simulink model "pattern3x3_testing_2023v1"  (R2023a)
settings: Solver=FixedStepAuto  StartTime=0.0  StopTime=2  FixedStep=0.000005  RelTol=1e-3
values from neighbouring files (symbols this model uses):
  test_pattern = load('Pattern4_test.CSV')    [model_setup_test.m]
  Th_control_time2 = 0.02    [model_setup4.m]    (also in model_setup_test.m = 2)
  Th_minus_count2 = 10    [model_setup4.m]    (also in model_setup_test.m = 5)
  Th_plus_count2 = 20    [model_setup4.m]    (also in model_setup_test.m)
libraries: simulink x1
(part 4 of 4)

== system pattern3x3_testing_2023v1/Synapse30/Spike_gererator ==
  "Spike " : Inport
  AND : Logic  IconShape=distinctive  AllPortsSameDT=off  OutDataTypeStr=boolean
  Delay : Delay  DelayLength=1  SampleTime=0.00001
  NOT : Logic  Operator=NOT  IconShape=distinctive  AllPortsSameDT=off  OutDataTypeStr=boolean
  Spike_out : Outport  VectorParamsAs1DForOutWhenUnconnected=off
  wires:
  "Spike "/1 -> NOT/1, AND/1
  AND/1 -> Spike_out/1
  Delay/1 -> AND/2
  NOT/1 -> Delay/1

== system pattern3x3_testing_2023v1/Synapse31/Spike_gererator ==
  "Spike " : Inport
  AND : Logic  IconShape=distinctive  AllPortsSameDT=off  OutDataTypeStr=boolean
  Delay : Delay  DelayLength=1  SampleTime=0.00001
  NOT : Logic  Operator=NOT  IconShape=distinctive  AllPortsSameDT=off  OutDataTypeStr=boolean
  Spike_out : Outport  VectorParamsAs1DForOutWhenUnconnected=off
  wires:
  "Spike "/1 -> NOT/1, AND/1
  AND/1 -> Spike_out/1
  Delay/1 -> AND/2
  NOT/1 -> Delay/1

== system pattern3x3_testing_2023v1/Synapse32/Spike_gererator ==
  "Spike " : Inport
  AND : Logic  IconShape=distinctive  AllPortsSameDT=off  OutDataTypeStr=boolean
  Delay : Delay  DelayLength=1  SampleTime=0.00001
  NOT : Logic  Operator=NOT  IconShape=distinctive  AllPortsSameDT=off  OutDataTypeStr=boolean
  Spike_out : Outport  VectorParamsAs1DForOutWhenUnconnected=off
  wires:
  "Spike "/1 -> NOT/1, AND/1
  AND/1 -> Spike_out/1
  Delay/1 -> AND/2
  NOT/1 -> Delay/1

== system pattern3x3_testing_2023v1/Synapse33/Spike_gererator ==
  "Spike " : Inport
  AND : Logic  IconShape=distinctive  AllPortsSameDT=off  OutDataTypeStr=boolean
  Delay : Delay  DelayLength=1  SampleTime=0.00001
  NOT : Logic  Operator=NOT  IconShape=distinctive  AllPortsSameDT=off  OutDataTypeStr=boolean
  Spike_out : Outport  VectorParamsAs1DForOutWhenUnconnected=off
  wires:
  "Spike "/1 -> NOT/1, AND/1
  AND/1 -> Spike_out/1
  Delay/1 -> AND/2
  NOT/1 -> Delay/1

== system pattern3x3_testing_2023v1/Synapse34/Spike_gererator ==
  "Spike " : Inport
  AND : Logic  IconShape=distinctive  AllPortsSameDT=off  OutDataTypeStr=boolean
  Delay : Delay  DelayLength=1  SampleTime=0.00001
  NOT : Logic  Operator=NOT  IconShape=distinctive  AllPortsSameDT=off  OutDataTypeStr=boolean
  Spike_out : Outport  VectorParamsAs1DForOutWhenUnconnected=off
  wires:
  "Spike "/1 -> NOT/1, AND/1
  AND/1 -> Spike_out/1
  Delay/1 -> AND/2
  NOT/1 -> Delay/1

== system pattern3x3_testing_2023v1/Synapse35/Spike_gererator ==
  "Spike " : Inport
  AND : Logic  IconShape=distinctive  AllPortsSameDT=off  OutDataTypeStr=boolean
  Delay : Delay  DelayLength=1  SampleTime=0.00001
  NOT : Logic  Operator=NOT  IconShape=distinctive  AllPortsSameDT=off  OutDataTypeStr=boolean
  Spike_out : Outport  VectorParamsAs1DForOutWhenUnconnected=off
  wires:
  "Spike "/1 -> NOT/1, AND/1
  AND/1 -> Spike_out/1
  Delay/1 -> AND/2
  NOT/1 -> Delay/1

== system pattern3x3_testing_2023v1/Synapse36/Spike_gererator ==
  "Spike " : Inport
  AND : Logic  IconShape=distinctive  AllPortsSameDT=off  OutDataTypeStr=boolean
  Delay : Delay  DelayLength=1  SampleTime=0.00001
  NOT : Logic  Operator=NOT  IconShape=distinctive  AllPortsSameDT=off  OutDataTypeStr=boolean
  Spike_out : Outport  VectorParamsAs1DForOutWhenUnconnected=off
  wires:
  "Spike "/1 -> NOT/1, AND/1
  AND/1 -> Spike_out/1
  Delay/1 -> AND/2
  NOT/1 -> Delay/1

== system pattern3x3_testing_2023v1/Synapse4/Spike_gererator ==
  "Spike " : Inport
  AND : Logic  IconShape=distinctive  AllPortsSameDT=off  OutDataTypeStr=boolean
  Delay : Delay  DelayLength=1  SampleTime=0.00001
  NOT : Logic  Operator=NOT  IconShape=distinctive  AllPortsSameDT=off  OutDataTypeStr=boolean
  Spike_out : Outport  VectorParamsAs1DForOutWhenUnconnected=off
  wires:
  "Spike "/1 -> NOT/1, AND/1
  AND/1 -> Spike_out/1
  Delay/1 -> AND/2
  NOT/1 -> Delay/1

== system pattern3x3_testing_2023v1/Synapse5/Spike_gererator ==
  "Spike " : Inport
  AND : Logic  IconShape=distinctive  AllPortsSameDT=off  OutDataTypeStr=boolean
  Delay : Delay  DelayLength=1  SampleTime=0.00001
  NOT : Logic  Operator=NOT  IconShape=distinctive  AllPortsSameDT=off  OutDataTypeStr=boolean
  Spike_out : Outport  VectorParamsAs1DForOutWhenUnconnected=off
  wires:
  "Spike "/1 -> NOT/1, AND/1
  AND/1 -> Spike_out/1
  Delay/1 -> AND/2
  NOT/1 -> Delay/1

== system pattern3x3_testing_2023v1/Synapse6/Spike_gererator ==
  "Spike " : Inport
  AND : Logic  IconShape=distinctive  AllPortsSameDT=off  OutDataTypeStr=boolean
  Delay : Delay  DelayLength=1  SampleTime=0.00001
  NOT : Logic  Operator=NOT  IconShape=distinctive  AllPortsSameDT=off  OutDataTypeStr=boolean
  Spike_out : Outport  VectorParamsAs1DForOutWhenUnconnected=off
  wires:
  "Spike "/1 -> NOT/1, AND/1
  AND/1 -> Spike_out/1
  Delay/1 -> AND/2
  NOT/1 -> Delay/1

== system pattern3x3_testing_2023v1/Synapse7/Spike_gererator ==
  "Spike " : Inport
  AND : Logic  IconShape=distinctive  AllPortsSameDT=off  OutDataTypeStr=boolean
  Delay : Delay  DelayLength=1  SampleTime=0.00001
  NOT : Logic  Operator=NOT  IconShape=distinctive  AllPortsSameDT=off  OutDataTypeStr=boolean
  Spike_out : Outport  VectorParamsAs1DForOutWhenUnconnected=off
  wires:
  "Spike "/1 -> NOT/1, AND/1
  AND/1 -> Spike_out/1
  Delay/1 -> AND/2
  NOT/1 -> Delay/1

== system pattern3x3_testing_2023v1/Synapse8/Spike_gererator ==
  "Spike " : Inport
  AND : Logic  IconShape=distinctive  AllPortsSameDT=off  OutDataTypeStr=boolean
  Delay : Delay  DelayLength=1  SampleTime=0.00001
  NOT : Logic  Operator=NOT  IconShape=distinctive  AllPortsSameDT=off  OutDataTypeStr=boolean
  Spike_out : Outport  VectorParamsAs1DForOutWhenUnconnected=off
  wires:
  "Spike "/1 -> NOT/1, AND/1
  AND/1 -> Spike_out/1
  Delay/1 -> AND/2
  NOT/1 -> Delay/1

== system pattern3x3_testing_2023v1/Synapse9/Spike_gererator ==
  "Spike " : Inport
  AND : Logic  IconShape=distinctive  AllPortsSameDT=off  OutDataTypeStr=boolean
  Delay : Delay  DelayLength=1  SampleTime=0.00001
  NOT : Logic  Operator=NOT  IconShape=distinctive  AllPortsSameDT=off  OutDataTypeStr=boolean
  Spike_out : Outport  VectorParamsAs1DForOutWhenUnconnected=off
  wires:
  "Spike "/1 -> NOT/1, AND/1
  AND/1 -> Spike_out/1
  Delay/1 -> AND/2
  NOT/1 -> Delay/1

== system pattern3x3_testing_2023v1/Neuron1/Clock4/Triggered Subsystem1 ==
  In1 : Inport
  Trigger : TriggerPort  VariantControl=Variant
  Constant : Constant
  Sum : Sum  Inputs=|++
  Out1 : Outport  VectorParamsAs1DForOutWhenUnconnected=off
  wires:
  Constant/1 -> Sum/2
  In1/1 -> Sum/1
  Sum/1 -> Out1/1

== system pattern3x3_testing_2023v1/Neuron1/Clock5/Triggered Subsystem1 ==
  In1 : Inport
  Trigger : TriggerPort  VariantControl=Variant
  Constant : Constant
  Sum : Sum  Inputs=|++
  Out1 : Outport  VectorParamsAs1DForOutWhenUnconnected=off
  wires:
  Constant/1 -> Sum/2
  In1/1 -> Sum/1
  Sum/1 -> Out1/1

== system pattern3x3_testing_2023v1/Neuron1/Subsystem3/spike_generator2 ==
  del_th : Inport
  AND : Logic  IconShape=distinctive  AllPortsSameDT=off  OutDataTypeStr=boolean
  Delay1 : Delay  DelayLength=1  SampleTime=0.00001
  NOT : Logic  Operator=NOT  IconShape=distinctive  AllPortsSameDT=off  OutDataTypeStr=boolean
  Product : Product
  del_th_spike : Outport
  wires:
  NOT/1 -> Delay1/1
  AND/1 -> Product/1
  Delay1/1 -> AND/2
  Product/1 -> del_th_spike/1
  del_th/1 -> AND/1, Product/2, NOT/1

== system pattern3x3_testing_2023v1/Neuron2/Clock4/Triggered Subsystem1 ==
  In1 : Inport
  Trigger : TriggerPort  VariantControl=Variant
  Constant : Constant
  Sum : Sum  Inputs=|++
  Out1 : Outport  VectorParamsAs1DForOutWhenUnconnected=off
  wires:
  Constant/1 -> Sum/2
  In1/1 -> Sum/1
  Sum/1 -> Out1/1

== system pattern3x3_testing_2023v1/Neuron2/Clock5/Triggered Subsystem1 ==
  In1 : Inport
  Trigger : TriggerPort  VariantControl=Variant
  Constant : Constant
  Sum : Sum  Inputs=|++
  Out1 : Outport  VectorParamsAs1DForOutWhenUnconnected=off
  wires:
  Constant/1 -> Sum/2
  In1/1 -> Sum/1
  Sum/1 -> Out1/1

== system pattern3x3_testing_2023v1/Neuron2/Subsystem3/spike_generator2 ==
  del_th : Inport
  AND : Logic  IconShape=distinctive  AllPortsSameDT=off  OutDataTypeStr=boolean
  Delay1 : Delay  DelayLength=1  SampleTime=0.00001
  NOT : Logic  Operator=NOT  IconShape=distinctive  AllPortsSameDT=off  OutDataTypeStr=boolean
  Product : Product
  del_th_spike : Outport
  wires:
  NOT/1 -> Delay1/1
  AND/1 -> Product/1
  Delay1/1 -> AND/2
  Product/1 -> del_th_spike/1
  del_th/1 -> AND/1, Product/2, NOT/1

== system pattern3x3_testing_2023v1/Neuron3/Clock4/Triggered Subsystem1 ==
  In1 : Inport
  Trigger : TriggerPort  VariantControl=Variant
  Constant : Constant
  Sum : Sum  Inputs=|++
  Out1 : Outport  VectorParamsAs1DForOutWhenUnconnected=off
  wires:
  Constant/1 -> Sum/2
  In1/1 -> Sum/1
  Sum/1 -> Out1/1

== system pattern3x3_testing_2023v1/Neuron3/Clock5/Triggered Subsystem1 ==
  In1 : Inport
  Trigger : TriggerPort  VariantControl=Variant
  Constant : Constant
  Sum : Sum  Inputs=|++
  Out1 : Outport  VectorParamsAs1DForOutWhenUnconnected=off
  wires:
  Constant/1 -> Sum/2
  In1/1 -> Sum/1
  Sum/1 -> Out1/1

== system pattern3x3_testing_2023v1/Neuron3/Subsystem3/spike_generator2 ==
  del_th : Inport
  AND : Logic  IconShape=distinctive  AllPortsSameDT=off  OutDataTypeStr=boolean
  Delay1 : Delay  DelayLength=1  SampleTime=0.00001
  NOT : Logic  Operator=NOT  IconShape=distinctive  AllPortsSameDT=off  OutDataTypeStr=boolean
  Product : Product
  del_th_spike : Outport
  wires:
  NOT/1 -> Delay1/1
  AND/1 -> Product/1
  Delay1/1 -> AND/2
  Product/1 -> del_th_spike/1
  del_th/1 -> AND/1, Product/2, NOT/1

== system pattern3x3_testing_2023v1/Neuron4/Clock4/Triggered Subsystem1 ==
  In1 : Inport
  Trigger : TriggerPort  VariantControl=Variant
  Constant : Constant
  Sum : Sum  Inputs=|++
  Out1 : Outport  VectorParamsAs1DForOutWhenUnconnected=off
  wires:
  Constant/1 -> Sum/2
  In1/1 -> Sum/1
  Sum/1 -> Out1/1

== system pattern3x3_testing_2023v1/Neuron4/Clock5/Triggered Subsystem1 ==
  In1 : Inport
  Trigger : TriggerPort  VariantControl=Variant
  Constant : Constant
  Sum : Sum  Inputs=|++
  Out1 : Outport  VectorParamsAs1DForOutWhenUnconnected=off
  wires:
  Constant/1 -> Sum/2
  In1/1 -> Sum/1
  Sum/1 -> Out1/1

== system pattern3x3_testing_2023v1/Neuron4/Subsystem3/spike_generator2 ==
  del_th : Inport
  AND : Logic  IconShape=distinctive  AllPortsSameDT=off  OutDataTypeStr=boolean
  Delay1 : Delay  DelayLength=1  SampleTime=0.00001
  NOT : Logic  Operator=NOT  IconShape=distinctive  AllPortsSameDT=off  OutDataTypeStr=boolean
  Product : Product
  del_th_spike : Outport
  wires:
  NOT/1 -> Delay1/1
  AND/1 -> Product/1
  Delay1/1 -> AND/2
  Product/1 -> del_th_spike/1
  del_th/1 -> AND/1, Product/2, NOT/1

== system pattern3x3_testing_2023v1/Neuron5/Clock4/Triggered Subsystem1 ==
  In1 : Inport
  Trigger : TriggerPort  VariantControl=Variant
  Constant : Constant
  Sum : Sum  Inputs=|++
  Out1 : Outport  VectorParamsAs1DForOutWhenUnconnected=off
  wires:
  Constant/1 -> Sum/2
  In1/1 -> Sum/1
  Sum/1 -> Out1/1

== system pattern3x3_testing_2023v1/Neuron5/Clock5/Triggered Subsystem1 ==
  In1 : Inport
  Trigger : TriggerPort  VariantControl=Variant
  Constant : Constant
  Sum : Sum  Inputs=|++
  Out1 : Outport  VectorParamsAs1DForOutWhenUnconnected=off
  wires:
  Constant/1 -> Sum/2
  In1/1 -> Sum/1
  Sum/1 -> Out1/1

== system pattern3x3_testing_2023v1/Neuron5/Subsystem3/spike_generator2 ==
  del_th : Inport
  AND : Logic  IconShape=distinctive  AllPortsSameDT=off  OutDataTypeStr=boolean
  Delay1 : Delay  DelayLength=1  SampleTime=0.00001
  NOT : Logic  Operator=NOT  IconShape=distinctive  AllPortsSameDT=off  OutDataTypeStr=boolean
  Product : Product
  del_th_spike : Outport
  wires:
  NOT/1 -> Delay1/1
  AND/1 -> Product/1
  Delay1/1 -> AND/2
  Product/1 -> del_th_spike/1
  del_th/1 -> AND/1, Product/2, NOT/1

== system pattern3x3_testing_2023v1/Neuron6/Clock4/Triggered Subsystem1 ==
  In1 : Inport
  Trigger : TriggerPort  VariantControl=Variant
  Constant : Constant
  Sum : Sum  Inputs=|++
  Out1 : Outport  VectorParamsAs1DForOutWhenUnconnected=off
  wires:
  Constant/1 -> Sum/2
  In1/1 -> Sum/1
  Sum/1 -> Out1/1

== system pattern3x3_testing_2023v1/Neuron6/Clock5/Triggered Subsystem1 ==
  In1 : Inport
  Trigger : TriggerPort  VariantControl=Variant
  Constant : Constant
  Sum : Sum  Inputs=|++
  Out1 : Outport  VectorParamsAs1DForOutWhenUnconnected=off
  wires:
  Constant/1 -> Sum/2
  In1/1 -> Sum/1
  Sum/1 -> Out1/1

== system pattern3x3_testing_2023v1/Neuron6/Subsystem3/spike_generator2 ==
  del_th : Inport
  AND : Logic  IconShape=distinctive  AllPortsSameDT=off  OutDataTypeStr=boolean
  Delay1 : Delay  DelayLength=1  SampleTime=0.00001
  NOT : Logic  Operator=NOT  IconShape=distinctive  AllPortsSameDT=off  OutDataTypeStr=boolean
  Product : Product
  del_th_spike : Outport
  wires:
  NOT/1 -> Delay1/1
  AND/1 -> Product/1
  Delay1/1 -> AND/2
  Product/1 -> del_th_spike/1
  del_th/1 -> AND/1, Product/2, NOT/1

== system pattern3x3_testing_2023v1/Neuron7/Clock4/Triggered Subsystem1 ==
  In1 : Inport
  Trigger : TriggerPort  VariantControl=Variant
  Constant : Constant
  Sum : Sum  Inputs=|++
  Out1 : Outport  VectorParamsAs1DForOutWhenUnconnected=off
  wires:
  Constant/1 -> Sum/2
  In1/1 -> Sum/1
  Sum/1 -> Out1/1

== system pattern3x3_testing_2023v1/Neuron7/Clock5/Triggered Subsystem1 ==
  In1 : Inport
  Trigger : TriggerPort  VariantControl=Variant
  Constant : Constant
  Sum : Sum  Inputs=|++
  Out1 : Outport  VectorParamsAs1DForOutWhenUnconnected=off
  wires:
  Constant/1 -> Sum/2
  In1/1 -> Sum/1
  Sum/1 -> Out1/1

== system pattern3x3_testing_2023v1/Neuron7/Subsystem3/spike_generator2 ==
  del_th : Inport
  AND : Logic  IconShape=distinctive  AllPortsSameDT=off  OutDataTypeStr=boolean
  Delay1 : Delay  DelayLength=1  SampleTime=0.00001
  NOT : Logic  Operator=NOT  IconShape=distinctive  AllPortsSameDT=off  OutDataTypeStr=boolean
  Product : Product
  del_th_spike : Outport
  wires:
  NOT/1 -> Delay1/1
  AND/1 -> Product/1
  Delay1/1 -> AND/2
  Product/1 -> del_th_spike/1
  del_th/1 -> AND/1, Product/2, NOT/1

== system pattern3x3_testing_2023v1/Neuron8/Clock4/Triggered Subsystem1 ==
  In1 : Inport
  Trigger : TriggerPort  VariantControl=Variant
  Constant : Constant
  Sum : Sum  Inputs=|++
  Out1 : Outport  VectorParamsAs1DForOutWhenUnconnected=off
  wires:
  Constant/1 -> Sum/2
  In1/1 -> Sum/1
  Sum/1 -> Out1/1

== system pattern3x3_testing_2023v1/Neuron8/Clock5/Triggered Subsystem1 ==
  In1 : Inport
  Trigger : TriggerPort  VariantControl=Variant
  Constant : Constant
  Sum : Sum  Inputs=|++
  Out1 : Outport  VectorParamsAs1DForOutWhenUnconnected=off
  wires:
  Constant/1 -> Sum/2
  In1/1 -> Sum/1
  Sum/1 -> Out1/1

== system pattern3x3_testing_2023v1/Neuron8/Subsystem3/spike_generator2 ==
  del_th : Inport
  AND : Logic  IconShape=distinctive  AllPortsSameDT=off  OutDataTypeStr=boolean
  Delay1 : Delay  DelayLength=1  SampleTime=0.00001
  NOT : Logic  Operator=NOT  IconShape=distinctive  AllPortsSameDT=off  OutDataTypeStr=boolean
  Product : Product
  del_th_spike : Outport
  wires:
  NOT/1 -> Delay1/1
  AND/1 -> Product/1
  Delay1/1 -> AND/2
  Product/1 -> del_th_spike/1
  del_th/1 -> AND/1, Product/2, NOT/1

== system pattern3x3_testing_2023v1/Neuron9/Clock4/Triggered Subsystem1 ==
  In1 : Inport
  Trigger : TriggerPort  VariantControl=Variant
  Constant : Constant
  Sum : Sum  Inputs=|++
  Out1 : Outport  VectorParamsAs1DForOutWhenUnconnected=off
  wires:
  Constant/1 -> Sum/2
  In1/1 -> Sum/1
  Sum/1 -> Out1/1

== system pattern3x3_testing_2023v1/Neuron9/Clock5/Triggered Subsystem1 ==
  In1 : Inport
  Trigger : TriggerPort  VariantControl=Variant
  Constant : Constant
  Sum : Sum  Inputs=|++
  Out1 : Outport  VectorParamsAs1DForOutWhenUnconnected=off
  wires:
  Constant/1 -> Sum/2
  In1/1 -> Sum/1
  Sum/1 -> Out1/1

== system pattern3x3_testing_2023v1/Neuron9/Subsystem3/spike_generator2 ==
  del_th : Inport
  AND : Logic  IconShape=distinctive  AllPortsSameDT=off  OutDataTypeStr=boolean
  Delay1 : Delay  DelayLength=1  SampleTime=0.00001
  NOT : Logic  Operator=NOT  IconShape=distinctive  AllPortsSameDT=off  OutDataTypeStr=boolean
  Product : Product
  del_th_spike : Outport
  wires:
  NOT/1 -> Delay1/1
  AND/1 -> Product/1
  Delay1/1 -> AND/2
  Product/1 -> del_th_spike/1
  del_th/1 -> AND/1, Product/2, NOT/1

== system pattern3x3_testing_2023v1/Post_Neuron1/Clock4/Triggered Subsystem1 ==
  In1 : Inport
  Trigger : TriggerPort  VariantControl=Variant
  Constant : Constant
  Sum : Sum  Inputs=|++
  Out1 : Outport  VectorParamsAs1DForOutWhenUnconnected=off
  wires:
  Constant/1 -> Sum/2
  In1/1 -> Sum/1
  Sum/1 -> Out1/1

== system pattern3x3_testing_2023v1/Post_Neuron1/Clock6/Triggered Subsystem1 ==
  In1 : Inport
  Trigger : TriggerPort  VariantControl=Variant
  Constant : Constant
  Sum : Sum  Inputs=|++
  Out1 : Outport  VectorParamsAs1DForOutWhenUnconnected=off
  wires:
  Constant/1 -> Sum/2
  In1/1 -> Sum/1
  Sum/1 -> Out1/1

== system pattern3x3_testing_2023v1/Post_Neuron1/Subsystem3/spike_generator2 ==
  del_th : Inport
  AND : Logic  IconShape=distinctive  AllPortsSameDT=off  OutDataTypeStr=boolean
  Delay1 : Delay  DelayLength=1  SampleTime=0.00001
  NOT : Logic  Operator=NOT  IconShape=distinctive  AllPortsSameDT=off  OutDataTypeStr=boolean
  Product : Product
  del_th_spike : Outport
  wires:
  NOT/1 -> Delay1/1
  AND/1 -> Product/1
  Delay1/1 -> AND/2
  Product/1 -> del_th_spike/1
  del_th/1 -> AND/1, Product/2, NOT/1

== system pattern3x3_testing_2023v1/Post_Neuron2/Clock4/Triggered Subsystem1 ==
  In1 : Inport
  Trigger : TriggerPort  VariantControl=Variant
  Constant : Constant
  Sum : Sum  Inputs=|++
  Out1 : Outport  VectorParamsAs1DForOutWhenUnconnected=off
  wires:
  Constant/1 -> Sum/2
  In1/1 -> Sum/1
  Sum/1 -> Out1/1

== system pattern3x3_testing_2023v1/Post_Neuron2/Clock6/Triggered Subsystem1 ==
  In1 : Inport
  Trigger : TriggerPort  VariantControl=Variant
  Constant : Constant
  Sum : Sum  Inputs=|++
  Out1 : Outport  VectorParamsAs1DForOutWhenUnconnected=off
  wires:
  Constant/1 -> Sum/2
  In1/1 -> Sum/1
  Sum/1 -> Out1/1

== system pattern3x3_testing_2023v1/Post_Neuron2/Subsystem3/spike_generator2 ==
  del_th : Inport
  AND : Logic  IconShape=distinctive  AllPortsSameDT=off  OutDataTypeStr=boolean
  Delay1 : Delay  DelayLength=1  SampleTime=0.00001
  NOT : Logic  Operator=NOT  IconShape=distinctive  AllPortsSameDT=off  OutDataTypeStr=boolean
  Product : Product
  del_th_spike : Outport
  wires:
  NOT/1 -> Delay1/1
  AND/1 -> Product/1
  Delay1/1 -> AND/2
  Product/1 -> del_th_spike/1
  del_th/1 -> AND/1, Product/2, NOT/1

== system pattern3x3_testing_2023v1/Post_Neuron3/Clock4/Triggered Subsystem1 ==
  In1 : Inport
  Trigger : TriggerPort  VariantControl=Variant
  Constant : Constant
  Sum : Sum  Inputs=|++
  Out1 : Outport  VectorParamsAs1DForOutWhenUnconnected=off
  wires:
  Constant/1 -> Sum/2
  In1/1 -> Sum/1
  Sum/1 -> Out1/1

== system pattern3x3_testing_2023v1/Post_Neuron3/Clock6/Triggered Subsystem1 ==
  In1 : Inport
  Trigger : TriggerPort  VariantControl=Variant
  Constant : Constant
  Sum : Sum  Inputs=|++
  Out1 : Outport  VectorParamsAs1DForOutWhenUnconnected=off
  wires:
  Constant/1 -> Sum/2
  In1/1 -> Sum/1
  Sum/1 -> Out1/1

== system pattern3x3_testing_2023v1/Post_Neuron3/Subsystem3/spike_generator2 ==
  del_th : Inport
  AND : Logic  IconShape=distinctive  AllPortsSameDT=off  OutDataTypeStr=boolean
  Delay1 : Delay  DelayLength=1  SampleTime=0.00001
  NOT : Logic  Operator=NOT  IconShape=distinctive  AllPortsSameDT=off  OutDataTypeStr=boolean
  Product : Product
  del_th_spike : Outport
  wires:
  NOT/1 -> Delay1/1
  AND/1 -> Product/1
  Delay1/1 -> AND/2
  Product/1 -> del_th_spike/1
  del_th/1 -> AND/1, Product/2, NOT/1

== system pattern3x3_testing_2023v1/Post_Neuron4/Clock4/Triggered Subsystem1 ==
  In1 : Inport
  Trigger : TriggerPort  VariantControl=Variant
  Constant : Constant
  Sum : Sum  Inputs=|++
  Out1 : Outport  VectorParamsAs1DForOutWhenUnconnected=off
  wires:
  Constant/1 -> Sum/2
  In1/1 -> Sum/1
  Sum/1 -> Out1/1

== system pattern3x3_testing_2023v1/Post_Neuron4/Clock6/Triggered Subsystem1 ==
  In1 : Inport
  Trigger : TriggerPort  VariantControl=Variant
  Constant : Constant
  Sum : Sum  Inputs=|++
  Out1 : Outport  VectorParamsAs1DForOutWhenUnconnected=off
  wires:
  Constant/1 -> Sum/2
  In1/1 -> Sum/1
  Sum/1 -> Out1/1

== system pattern3x3_testing_2023v1/Post_Neuron4/Subsystem3/spike_generator2 ==
  del_th : Inport
  AND : Logic  IconShape=distinctive  AllPortsSameDT=off  OutDataTypeStr=boolean
  Delay1 : Delay  DelayLength=1  SampleTime=0.00001
  NOT : Logic  Operator=NOT  IconShape=distinctive  AllPortsSameDT=off  OutDataTypeStr=boolean
  Product : Product
  del_th_spike : Outport
  wires:
  NOT/1 -> Delay1/1
  AND/1 -> Product/1
  Delay1/1 -> AND/2
  Product/1 -> del_th_spike/1
  del_th/1 -> AND/1, Product/2, NOT/1

== matlab function pattern3x3_testing_2023v1/Neuron4/MATLAB Function3 ==
  data: u input; y output
function y = fcn(u)

if u>=0
    y=1;
else
    y=0;
end

== matlab function pattern3x3_testing_2023v1/Neuron4/MATLAB Function4 ==
  data: membrane_state input; t input; membrane_potential output
function membrane_potential = fcn(membrane_state, t)

membrane_potential = (membrane_state) * (exp(-(t)*0.015));

== matlab function pattern3x3_testing_2023v1/Neuron2/MATLAB Function3 ==
  data: u input; y output
function y = fcn(u)

if u>=0
    y=1;
else
    y=0;
end

== matlab function pattern3x3_testing_2023v1/Neuron4/MATLAB Function5 ==
  data: t input; membrane_state input; membrane_potential output
function membrane_potential = fcn(t, membrane_state)

membrane_potential = (membrane_state) * 2.361128*(exp(-(t)*0.09)-0.6*exp(-(t+1)*0.04)) ;

== matlab function pattern3x3_testing_2023v1/Neuron4/Subsystem3/MATLAB Function ==
  data: u input; y output; min input; max input
function y = fcn(u, min, max)

if u<=min
    y=min;
elseif u>=max
    y=max;
else
    y=u;
end

== matlab function pattern3x3_testing_2023v1/Neuron4/Subsystem3/MATLAB Function2 ==
  data: init_th input; y output; neuron_num input; before_threshold input
function y = fcn(init_th, neuron_num, before_threshold)

persistent n;

if isempty(n)
    n=init_th(neuron_num);
else
    n=before_threshold;
end

y=n;

== matlab function pattern3x3_testing_2023v1/Neuron5/MATLAB Function3 ==
  data: u input; y output
function y = fcn(u)

if u>=0
    y=1;
else
    y=0;
end

== matlab function pattern3x3_testing_2023v1/Neuron5/MATLAB Function4 ==
  data: membrane_state input; t input; membrane_potential output
function membrane_potential = fcn(membrane_state, t)

membrane_potential = (membrane_state) * (exp(-(t)*0.015));

== matlab function pattern3x3_testing_2023v1/Neuron5/MATLAB Function5 ==
  data: t input; membrane_state input; membrane_potential output
function membrane_potential = fcn(t, membrane_state)

membrane_potential = (membrane_state) * 2.361128*(exp(-(t)*0.09)-0.6*exp(-(t+1)*0.04)) ;

== matlab function pattern3x3_testing_2023v1/Neuron5/Subsystem3/MATLAB Function ==
  data: u input; y output; min input; max input
function y = fcn(u, min, max)

if u<=min
    y=min;
elseif u>=max
    y=max;
else
    y=u;
end

== matlab function pattern3x3_testing_2023v1/Neuron5/Subsystem3/MATLAB Function2 ==
  data: init_th input; y output; neuron_num input; before_threshold input
function y = fcn(init_th, neuron_num, before_threshold)

persistent n;

if isempty(n)
    n=init_th(neuron_num);
else
    n=before_threshold;
end

y=n;

== matlab function pattern3x3_testing_2023v1/Neuron2/MATLAB Function4 ==
  data: membrane_state input; t input; membrane_potential output
function membrane_potential = fcn(membrane_state, t)

membrane_potential = (membrane_state) * (exp(-(t)*0.015));

== matlab function pattern3x3_testing_2023v1/Neuron6/MATLAB Function3 ==
  data: u input; y output
function y = fcn(u)

if u>=0
    y=1;
else
    y=0;
end

== matlab function pattern3x3_testing_2023v1/Neuron6/MATLAB Function4 ==
  data: membrane_state input; t input; membrane_potential output
function membrane_potential = fcn(membrane_state, t)

membrane_potential = (membrane_state) * (exp(-(t)*0.015));

== matlab function pattern3x3_testing_2023v1/Neuron6/MATLAB Function5 ==
  data: t input; membrane_state input; membrane_potential output
function membrane_potential = fcn(t, membrane_state)

membrane_potential = (membrane_state) * 2.361128*(exp(-(t)*0.09)-0.6*exp(-(t+1)*0.04)) ;

== matlab function pattern3x3_testing_2023v1/Post_Neuron2/MATLAB Function3 ==
  data: membrane_state input; t input; membrane_potential output
function membrane_potential = fcn(membrane_state, t)

membrane_potential = (membrane_state) * (exp(-(t)*0.015));

== matlab function pattern3x3_testing_2023v1/Post_Neuron2/MATLAB Function4 ==
  data: t input; membrane_state input; membrane_potential output
function membrane_potential = fcn(t, membrane_state)

membrane_potential = (membrane_state) * 2.361128*(exp(-(t)*0.09)-0.6*exp(-(t+1)*0.04)) ;

== matlab function pattern3x3_testing_2023v1/Post_Neuron2/MATLAB Function7 ==
  data: rc input; lateral_inhibition input; t input; inhibition_potential output
function inhibition_potential = fcn(rc, lateral_inhibition, t)

inhibition_potential = -lateral_inhibition * (exp(-(t)*rc));

== matlab function pattern3x3_testing_2023v1/Post_Neuron2/Subsystem3/MATLAB Function ==
  data: u input; y output; min input; max input
function y = fcn(u, min, max)

if u<=min
    y=min;
elseif u>=max
    y=max;
else
    y=u;
end

== matlab function pattern3x3_testing_2023v1/Post_Neuron2/Subsystem3/MATLAB Function2 ==
  data: init_th input; y output; neuron_num input; before_threshold input
function y = fcn(init_th, neuron_num, before_threshold)

persistent n;

if isempty(n)
    n=init_th(neuron_num);
else
    n=before_threshold;
end

y=n;

== matlab function pattern3x3_testing_2023v1/Post_Neuron3/MATLAB Function1 ==
  data: u input; y output
function y = fcn(u)

if u>=0
    y=1;
else
    y=0;
end

== matlab function pattern3x3_testing_2023v1/Post_Neuron3/MATLAB Function2 ==
  data: u input; y output
function y = fcn(u)
persistent k;
if isempty(k)
    k=0;
elseif u>0
    k=1;
end

y=k;

== matlab function pattern3x3_testing_2023v1/Neuron2/MATLAB Function5 ==
  data: t input; membrane_state input; membrane_potential output
function membrane_potential = fcn(t, membrane_state)

membrane_potential = (membrane_state) * 2.361128*(exp(-(t)*0.09)-0.6*exp(-(t+1)*0.04)) ;

== matlab function pattern3x3_testing_2023v1/Post_Neuron3/MATLAB Function3 ==
  data: membrane_state input; t input; membrane_potential output
function membrane_potential = fcn(membrane_state, t)

membrane_potential = (membrane_state) * (exp(-(t)*0.015));

== matlab function pattern3x3_testing_2023v1/Post_Neuron3/MATLAB Function4 ==
  data: t input; membrane_state input; membrane_potential output
function membrane_potential = fcn(t, membrane_state)

membrane_potential = (membrane_state) * 2.361128*(exp(-(t)*0.09)-0.6*exp(-(t+1)*0.04)) ;

== matlab function pattern3x3_testing_2023v1/Post_Neuron3/MATLAB Function7 ==
  data: rc input; lateral_inhibition input; t input; inhibition_potential output
function inhibition_potential = fcn(rc, lateral_inhibition, t)

inhibition_potential = -lateral_inhibition * (exp(-(t)*rc));

== matlab function pattern3x3_testing_2023v1/Neuron6/Subsystem3/MATLAB Function ==
  data: u input; y output; min input; max input
function y = fcn(u, min, max)

if u<=min
    y=min;
elseif u>=max
    y=max;
else
    y=u;
end

== matlab function pattern3x3_testing_2023v1/Neuron6/Subsystem3/MATLAB Function2 ==
  data: init_th input; y output; neuron_num input; before_threshold input
function y = fcn(init_th, neuron_num, before_threshold)

persistent n;

if isempty(n)
    n=init_th(neuron_num);
else
    n=before_threshold;
end

y=n;

== matlab function pattern3x3_testing_2023v1/Post_Neuron3/Subsystem3/MATLAB Function ==
  data: u input; y output; min input; max input
function y = fcn(u, min, max)

if u<=min
    y=min;
elseif u>=max
    y=max;
else
    y=u;
end

== matlab function pattern3x3_testing_2023v1/Post_Neuron3/Subsystem3/MATLAB Function2 ==
  data: init_th input; y output; neuron_num input; before_threshold input
function y = fcn(init_th, neuron_num, before_threshold)

persistent n;

if isempty(n)
    n=init_th(neuron_num);
else
    n=before_threshold;
end

y=n;

== matlab function pattern3x3_testing_2023v1/Post_Neuron4/MATLAB Function1 ==
  data: u input; y output
function y = fcn(u)

if u>=0
    y=1;
else
    y=0;
end

== matlab function pattern3x3_testing_2023v1/Synapse2/MATLAB Function1 ==
  data: y output; syna_var input; addr input
function y = fcn(syna_var,addr)


   
        y=syna_var(addr);
    

end

== matlab function pattern3x3_testing_2023v1/Synapse3/MATLAB Function1 ==
  data: y output; syna_var input; addr input
function y = fcn(syna_var,addr)


   
        y=syna_var(addr);
    

end

== matlab function pattern3x3_testing_2023v1/Post_Neuron2/MATLAB Function1 ==
  data: u input; y output
function y = fcn(u)

if u>=0
    y=1;
else
    y=0;
end

== matlab function pattern3x3_testing_2023v1/Synapse4/MATLAB Function1 ==
  data: y output; syna_var input; addr input
function y = fcn(syna_var,addr)


   
        y=syna_var(addr);
    

end

== matlab function pattern3x3_testing_2023v1/Synapse5/MATLAB Function1 ==
  data: y output; syna_var input; addr input
function y = fcn(syna_var,addr)


   
        y=syna_var(addr);
    

end

== matlab function pattern3x3_testing_2023v1/Synapse6/MATLAB Function1 ==
  data: y output; syna_var input; addr input
function y = fcn(syna_var,addr)


   
        y=syna_var(addr);
    

end

== matlab function pattern3x3_testing_2023v1/Synapse7/MATLAB Function1 ==
  data: y output; syna_var input; addr input
function y = fcn(syna_var,addr)


   
        y=syna_var(addr);
    

end

== matlab function pattern3x3_testing_2023v1/Synapse8/MATLAB Function1 ==
  data: y output; syna_var input; addr input
function y = fcn(syna_var,addr)


   
        y=syna_var(addr);
    

end

== matlab function pattern3x3_testing_2023v1/Synapse9/MATLAB Function1 ==
  data: y output; syna_var input; addr input
function y = fcn(syna_var,addr)


   
        y=syna_var(addr);
    

end

== matlab function pattern3x3_testing_2023v1/Synapse10/MATLAB Function1 ==
  data: y output; syna_var input; addr input
function y = fcn(syna_var,addr)


   
        y=syna_var(addr);
    

end

== matlab function pattern3x3_testing_2023v1/Synapse11/MATLAB Function1 ==
  data: y output; syna_var input; addr input
function y = fcn(syna_var,addr)


   
        y=syna_var(addr);
    

end

== matlab function pattern3x3_testing_2023v1/Synapse12/MATLAB Function1 ==
  data: y output; syna_var input; addr input
function y = fcn(syna_var,addr)


   
        y=syna_var(addr);
    

end

== matlab function pattern3x3_testing_2023v1/Post_Neuron2/MATLAB Function2 ==
  data: u input; y output
function y = fcn(u)
persistent k;
if isempty(k)
    k=0;
elseif u>0
    k=1;
end

y=k;

== matlab function pattern3x3_testing_2023v1/Synapse13/MATLAB Function1 ==
  data: y output; syna_var input; addr input
function y = fcn(syna_var,addr)


   
        y=syna_var(addr);
    

end

== matlab function pattern3x3_testing_2023v1/Synapse14/MATLAB Function1 ==
  data: y output; syna_var input; addr input
function y = fcn(syna_var,addr)


   
        y=syna_var(addr);
    

end

== matlab function pattern3x3_testing_2023v1/Synapse15/MATLAB Function1 ==
  data: y output; syna_var input; addr input
function y = fcn(syna_var,addr)


   
        y=syna_var(addr);
    

end

== matlab function pattern3x3_testing_2023v1/Synapse16/MATLAB Function1 ==
  data: y output; syna_var input; addr input
function y = fcn(syna_var,addr)


   
        y=syna_var(addr);
    

end

== matlab function pattern3x3_testing_2023v1/Synapse17/MATLAB Function1 ==
  data: y output; syna_var input; addr input
function y = fcn(syna_var,addr)


   
        y=syna_var(addr);
    

end

== matlab function pattern3x3_testing_2023v1/Synapse18/MATLAB Function1 ==
  data: y output; syna_var input; addr input
function y = fcn(syna_var,addr)


   
        y=syna_var(addr);
    

end

== matlab function pattern3x3_testing_2023v1/Synapse19/MATLAB Function1 ==
  data: y output; syna_var input; addr input
function y = fcn(syna_var,addr)


   
        y=syna_var(addr);
    

end

== matlab function pattern3x3_testing_2023v1/Synapse20/MATLAB Function1 ==
  data: y output; syna_var input; addr input
function y = fcn(syna_var,addr)


   
        y=syna_var(addr);
    

end

== matlab function pattern3x3_testing_2023v1/Neuron2/Subsystem3/MATLAB Function ==
  data: u input; y output; min input; max input
function y = fcn(u, min, max)

if u<=min
    y=min;
elseif u>=max
    y=max;
else
    y=u;
end

== matlab function pattern3x3_testing_2023v1/Synapse21/MATLAB Function1 ==
  data: y output; syna_var input; addr input
function y = fcn(syna_var,addr)


   
        y=syna_var(addr);
    

end

== matlab function pattern3x3_testing_2023v1/Synapse22/MATLAB Function1 ==
  data: y output; syna_var input; addr input
function y = fcn(syna_var,addr)


   
        y=syna_var(addr);
    

end

== matlab function pattern3x3_testing_2023v1/Synapse23/MATLAB Function1 ==
  data: y output; syna_var input; addr input
function y = fcn(syna_var,addr)


   
        y=syna_var(addr);
    

end

== matlab function pattern3x3_testing_2023v1/Synapse24/MATLAB Function1 ==
  data: y output; syna_var input; addr input
function y = fcn(syna_var,addr)


   
        y=syna_var(addr);
    

end

== matlab function pattern3x3_testing_2023v1/Synapse25/MATLAB Function1 ==
  data: y output; syna_var input; addr input
function y = fcn(syna_var,addr)


   
        y=syna_var(addr);
    

end

== matlab function pattern3x3_testing_2023v1/Synapse26/MATLAB Function1 ==
  data: y output; syna_var input; addr input
function y = fcn(syna_var,addr)


   
        y=syna_var(addr);
    

end

== matlab function pattern3x3_testing_2023v1/Synapse27/MATLAB Function1 ==
  data: y output; syna_var input; addr input
function y = fcn(syna_var,addr)


   
        y=syna_var(addr);
    

end

== matlab function pattern3x3_testing_2023v1/Synapse28/MATLAB Function1 ==
  data: y output; syna_var input; addr input
function y = fcn(syna_var,addr)


   
        y=syna_var(addr);
    

end

== matlab function pattern3x3_testing_2023v1/Synapse29/MATLAB Function1 ==
  data: y output; syna_var input; addr input
function y = fcn(syna_var,addr)


   
        y=syna_var(addr);
    

end

== matlab function pattern3x3_testing_2023v1/Synapse30/MATLAB Function1 ==
  data: y output; syna_var input; addr input
function y = fcn(syna_var,addr)


   
        y=syna_var(addr);
    

end

== matlab function pattern3x3_testing_2023v1/Synapse31/MATLAB Function1 ==
  data: y output; syna_var input; addr input
function y = fcn(syna_var,addr)


   
        y=syna_var(addr);
    

end

== matlab function pattern3x3_testing_2023v1/Synapse32/MATLAB Function1 ==
  data: y output; syna_var input; addr input
function y = fcn(syna_var,addr)


   
        y=syna_var(addr);
    

end

== matlab function pattern3x3_testing_2023v1/Neuron2/Subsystem3/MATLAB Function2 ==
  data: init_th input; y output; neuron_num input; before_threshold input
function y = fcn(init_th, neuron_num, before_threshold)

persistent n;

if isempty(n)
    n=init_th(neuron_num);
else
    n=before_threshold;
end

y=n;

== matlab function pattern3x3_testing_2023v1/Synapse33/MATLAB Function1 ==
  data: y output; syna_var input; addr input
function y = fcn(syna_var,addr)


   
        y=syna_var(addr);
    

end

== matlab function pattern3x3_testing_2023v1/Synapse34/MATLAB Function1 ==
  data: y output; syna_var input; addr input
function y = fcn(syna_var,addr)


   
        y=syna_var(addr);
    

end

== matlab function pattern3x3_testing_2023v1/Synapse35/MATLAB Function1 ==
  data: y output; syna_var input; addr input
function y = fcn(syna_var,addr)


   
        y=syna_var(addr);
    

end

== matlab function pattern3x3_testing_2023v1/Synapse36/MATLAB Function1 ==
  data: y output; syna_var input; addr input
function y = fcn(syna_var,addr)


   
        y=syna_var(addr);
    

end

== matlab function pattern3x3_testing_2023v1/Post_Neuron4/MATLAB Function2 ==
  data: u input; y output
function y = fcn(u)
persistent k;
if isempty(k)
    k=0;
elseif u>0
    k=1;
end

y=k;

== matlab function pattern3x3_testing_2023v1/Post_Neuron4/MATLAB Function3 ==
  data: membrane_state input; t input; membrane_potential output
function membrane_potential = fcn(membrane_state, t)

membrane_potential = (membrane_state) * (exp(-(t)*0.015));

== matlab function pattern3x3_testing_2023v1/Post_Neuron4/MATLAB Function4 ==
  data: t input; membrane_state input; membrane_potential output
function membrane_potential = fcn(t, membrane_state)

membrane_potential = (membrane_state) * 2.361128*(exp(-(t)*0.09)-0.6*exp(-(t+1)*0.04)) ;

== matlab function pattern3x3_testing_2023v1/Post_Neuron4/MATLAB Function7 ==
  data: rc input; lateral_inhibition input; t input; inhibition_potential output
function inhibition_potential = fcn(rc, lateral_inhibition, t)

inhibition_potential = -lateral_inhibition * (exp(-(t)*rc));

== matlab function pattern3x3_testing_2023v1/Post_Neuron4/Subsystem3/MATLAB Function ==
  data: u input; y output; min input; max input
function y = fcn(u, min, max)

if u<=min
    y=min;
elseif u>=max
    y=max;
else
    y=u;
end

== matlab function pattern3x3_testing_2023v1/Post_Neuron4/Subsystem3/MATLAB Function2 ==
  data: init_th input; y output; neuron_num input; before_threshold input
function y = fcn(init_th, neuron_num, before_threshold)

persistent n;

if isempty(n)
    n=init_th(neuron_num);
else
    n=before_threshold;
end

y=n;

== matlab function pattern3x3_testing_2023v1/Neuron7/MATLAB Function3 ==
  data: u input; y output
function y = fcn(u)

if u>=0
    y=1;
else
    y=0;
end

== matlab function pattern3x3_testing_2023v1/Neuron3/MATLAB Function3 ==
  data: u input; y output
function y = fcn(u)

if u>=0
    y=1;
else
    y=0;
end

== matlab function pattern3x3_testing_2023v1/Neuron7/MATLAB Function4 ==
  data: membrane_state input; t input; membrane_potential output
function membrane_potential = fcn(membrane_state, t)

membrane_potential = (membrane_state) * (exp(-(t)*0.015));

== matlab function pattern3x3_testing_2023v1/Neuron7/MATLAB Function5 ==
  data: t input; membrane_state input; membrane_potential output
function membrane_potential = fcn(t, membrane_state)

membrane_potential = (membrane_state) * 2.361128*(exp(-(t)*0.09)-0.6*exp(-(t+1)*0.04)) ;

== matlab function pattern3x3_testing_2023v1/Neuron7/Subsystem3/MATLAB Function ==
  data: u input; y output; min input; max input
function y = fcn(u, min, max)

if u<=min
    y=min;
elseif u>=max
    y=max;
else
    y=u;
end

== matlab function pattern3x3_testing_2023v1/Neuron7/Subsystem3/MATLAB Function2 ==
  data: init_th input; y output; neuron_num input; before_threshold input
function y = fcn(init_th, neuron_num, before_threshold)

persistent n;

if isempty(n)
    n=init_th(neuron_num);
else
    n=before_threshold;
end

y=n;

== matlab function pattern3x3_testing_2023v1/Neuron8/MATLAB Function3 ==
  data: u input; y output
function y = fcn(u)

if u>=0
    y=1;
else
    y=0;
end

== matlab function pattern3x3_testing_2023v1/Neuron8/MATLAB Function4 ==
  data: membrane_state input; t input; membrane_potential output
function membrane_potential = fcn(membrane_state, t)

membrane_potential = (membrane_state) * (exp(-(t)*0.015));

== matlab function pattern3x3_testing_2023v1/Neuron8/MATLAB Function5 ==
  data: t input; membrane_state input; membrane_potential output
function membrane_potential = fcn(t, membrane_state)

membrane_potential = (membrane_state) * 2.361128*(exp(-(t)*0.09)-0.6*exp(-(t+1)*0.04)) ;

== matlab function pattern3x3_testing_2023v1/Neuron8/Subsystem3/MATLAB Function ==
  data: u input; y output; min input; max input
function y = fcn(u, min, max)

if u<=min
    y=min;
elseif u>=max
    y=max;
else
    y=u;
end

== matlab function pattern3x3_testing_2023v1/Neuron3/MATLAB Function4 ==
  data: membrane_state input; t input; membrane_potential output
function membrane_potential = fcn(membrane_state, t)

membrane_potential = (membrane_state) * (exp(-(t)*0.015));

== matlab function pattern3x3_testing_2023v1/Neuron8/Subsystem3/MATLAB Function2 ==
  data: init_th input; y output; neuron_num input; before_threshold input
function y = fcn(init_th, neuron_num, before_threshold)

persistent n;

if isempty(n)
    n=init_th(neuron_num);
else
    n=before_threshold;
end

y=n;

== matlab function pattern3x3_testing_2023v1/Neuron9/MATLAB Function3 ==
  data: u input; y output
function y = fcn(u)

if u>=0
    y=1;
else
    y=0;
end

== matlab function pattern3x3_testing_2023v1/Neuron9/MATLAB Function4 ==
  data: membrane_state input; t input; membrane_potential output
function membrane_potential = fcn(membrane_state, t)

membrane_potential = (membrane_state) * (exp(-(t)*0.015));

== matlab function pattern3x3_testing_2023v1/Neuron9/MATLAB Function5 ==
  data: t input; membrane_state input; membrane_potential output
function membrane_potential = fcn(t, membrane_state)

membrane_potential = (membrane_state) * 2.361128*(exp(-(t)*0.09)-0.6*exp(-(t+1)*0.04)) ;

== matlab function pattern3x3_testing_2023v1/Neuron9/Subsystem3/MATLAB Function ==
  data: u input; y output; min input; max input
function y = fcn(u, min, max)

if u<=min
    y=min;
elseif u>=max
    y=max;
else
    y=u;
end

== matlab function pattern3x3_testing_2023v1/Neuron9/Subsystem3/MATLAB Function2 ==
  data: init_th input; y output; neuron_num input; before_threshold input
function y = fcn(init_th, neuron_num, before_threshold)

persistent n;

if isempty(n)
    n=init_th(neuron_num);
else
    n=before_threshold;
end

y=n;

== matlab function pattern3x3_testing_2023v1/Post_Neuron1/MATLAB Function2 ==
  data: u input; y output
function y = fcn(u)
persistent k;
if isempty(k)
    k=0;
elseif u>0
    k=1;
end

y=k;

== matlab function pattern3x3_testing_2023v1/Post_Neuron1/MATLAB Function1 ==
  data: u input; y output
function y = fcn(u)

if u>=0
    y=1;
else
    y=0;
end

== matlab function pattern3x3_testing_2023v1/Post_Neuron1/MATLAB Function3 ==
  data: membrane_state input; t input; membrane_potential output
function membrane_potential = fcn(membrane_state, t)

membrane_potential = (membrane_state) * (exp(-(t)*0.015));

== matlab function pattern3x3_testing_2023v1/Post_Neuron1/MATLAB Function4 ==
  data: t input; membrane_state input; membrane_potential output
function membrane_potential = fcn(t, membrane_state)

membrane_potential = (membrane_state) * 2.361128*(exp(-(t)*0.09)-0.6*exp(-(t+1)*0.04)) ;

== matlab function pattern3x3_testing_2023v1/Neuron3/MATLAB Function5 ==
  data: t input; membrane_state input; membrane_potential output
function membrane_potential = fcn(t, membrane_state)

membrane_potential = (membrane_state) * 2.361128*(exp(-(t)*0.09)-0.6*exp(-(t+1)*0.04)) ;

== matlab function pattern3x3_testing_2023v1/Neuron1/MATLAB Function3 ==
  data: u input; y output
function y = fcn(u)

if u>=0
    y=1;
else
    y=0;
end

== matlab function pattern3x3_testing_2023v1/Post_Neuron1/Subsystem3/MATLAB Function ==
  data: u input; y output; min input; max input
function y = fcn(u, min, max)

if u<=min
    y=min;
elseif u>=max
    y=max;
else
    y=u;
end

== matlab function pattern3x3_testing_2023v1/Post_Neuron1/Subsystem3/MATLAB Function2 ==
  data: init_th input; y output; neuron_num input; before_threshold input
function y = fcn(init_th, neuron_num, before_threshold)

persistent n;

if isempty(n)
    n=init_th(neuron_num);
else
    n=before_threshold;
end

y=n;

== matlab function pattern3x3_testing_2023v1/Post_Neuron1/MATLAB Function7 ==
  data: rc input; lateral_inhibition input; t input; inhibition_potential output
function inhibition_potential = fcn(rc, lateral_inhibition, t)

inhibition_potential = -lateral_inhibition * (exp(-(t)*rc));

== matlab function pattern3x3_testing_2023v1/Neuron1/MATLAB Function4 ==
  data: membrane_state input; t input; membrane_potential output
function membrane_potential = fcn(membrane_state, t)

membrane_potential = (membrane_state) * (exp(-(t)*0.015));

== matlab function pattern3x3_testing_2023v1/Neuron1/MATLAB Function5 ==
  data: t input; membrane_state input; membrane_potential output
function membrane_potential = fcn(t, membrane_state)

membrane_potential = (membrane_state) * 2.361128*(exp(-(t)*0.09)-0.6*exp(-(t+1)*0.04)) ;

== matlab function pattern3x3_testing_2023v1/Neuron1/Subsystem3/MATLAB Function ==
  data: u input; y output; min input; max input
function y = fcn(u, min, max)

if u<=min
    y=min;
elseif u>=max
    y=max;
else
    y=u;
end

== matlab function pattern3x3_testing_2023v1/Neuron1/Subsystem3/MATLAB Function2 ==
  data: init_th input; y output; neuron_num input; before_threshold input
function y = fcn(init_th, neuron_num, before_threshold)

persistent n;

if isempty(n)
    n=init_th(neuron_num);
else
    n=before_threshold;
end

y=n;

== matlab function pattern3x3_testing_2023v1/Subsystem1/MATLAB Function ==
  data: data input; y output; i input
function y = fcn(data, i)

j=1+i;
 y=data(j,:);
          

   
end

== matlab function pattern3x3_testing_2023v1/Synapse1/MATLAB Function1 ==
  data: y output; syna_var input; addr input
function y = fcn(syna_var,addr)


   
        y=syna_var(addr);
    

end

== matlab function pattern3x3_testing_2023v1/Neuron3/Subsystem3/MATLAB Function ==
  data: u input; y output; min input; max input
function y = fcn(u, min, max)

if u<=min
    y=min;
elseif u>=max
    y=max;
else
    y=u;
end

== matlab function pattern3x3_testing_2023v1/Neuron3/Subsystem3/MATLAB Function2 ==
  data: init_th input; y output; neuron_num input; before_threshold input
function y = fcn(init_th, neuron_num, before_threshold)

persistent n;

if isempty(n)
    n=init_th(neuron_num);
else
    n=before_threshold;
end

y=n;
